simulink model "Expnserver_Model"  (R2024b)
settings: Solver=VariableStepAuto  StartTime=0.0  StopTime=10.0  RelTol=1e-3
libraries: NSA_DEVS_SINKS x4, NSA_DEVS_LOGISTICS x3, NSA_DEVS_SOURCES x1
settings Model: Creator=david  LastModifiedBy=peter
settings RTWCC: GPUComputeCapability=3.5

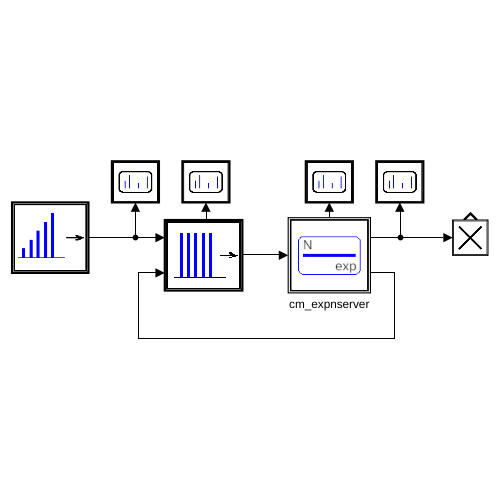
[thumbnail: Simulink's stored preview of the top-level diagram]
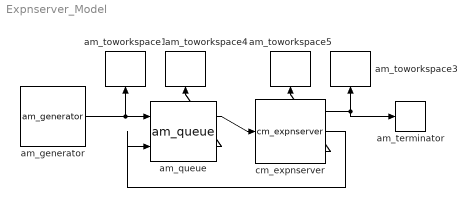
== system Expnserver_Model ==
  am_generator : NSA_DEVS_SOURCES/am_generator  tG=1  n0=1  nG=10  tD=[0,2]  debug=0
      settings: SourceProductName=Sources
  am_queue : NSA_DEVS_LOGISTICS/am_queue  tD=[0,2]  tau=[0,1]  debug=0
      settings: SourceProductName=Logistics
  am_terminator : NSA_DEVS_LOGISTICS/am_terminator  tau=[0,1]  debug=0
      settings: SourceProductName=Logistics
  am_toworkspace1 : NSA_DEVS_SINKS/am_toworkspace  varname="\"genOut\""  t0=0  format="\"vector\""  tau=[0,3]  debug=0
      settings: SourceProductName=Sinks
  am_toworkspace3 : NSA_DEVS_SINKS/am_toworkspace  varname="\"srvOut\""  t0=0  format="\"vector\""  tau=[0,3]  debug=0
      settings: SourceProductName=Sinks
  am_toworkspace4 : NSA_DEVS_SINKS/am_toworkspace  varname="\"nqOut\""  t0=0  format="\"vector\""  tau=[0,3]  debug=0
      settings: SourceProductName=Sinks
  am_toworkspace5 : NSA_DEVS_SINKS/am_toworkspace  varname="\"nsOut\""  t0=0  format="\"vector\""  tau=[0,5]  debug=0
      settings: SourceProductName=Sinks
  cm_expnserver : NSA_DEVS_LOGISTICS/cm_expnserver  N=3  tS=2.8  fieldname="\"serviceTime\""  tD=[0,2]  tau=[0,1]  debug=0
      settings: SourceProductName=Logistics
  wires:
  am_generator/1 -> am_queue/1, am_toworkspace1/1
  cm_expnserver/1 -> am_terminator/1, am_toworkspace3/1
  am_queue/1 -> cm_expnserver/1
  am_queue/2 -> am_toworkspace4/1
  cm_expnserver/3 -> am_toworkspace5/1
  cm_expnserver/2 -> am_queue/2
